simulink model "sdofDAEll_with_memory"  (R2023a)
settings: Solver=ode4  StartTime=0.0  StopTime=tmax  FixedStep=dt  RelTol=1e-3
InitFcn:
  | script_llm
values from neighbouring files (symbols this model uses):
  A1 = [O,I;-M1\K1,-M1\C1]    [script_llm.m]
  A2 = [O,I;-M2\K2,-M2\C2]    [script_llm.m]
  B1 = [0;0;M1\[0;1]]    [script_llm.m]
  B1b = -1    [script_llm.m]
  B2 = [0;0;M2\[0;1]]    [script_llm.m]
  B2b = -1    [script_llm.m]
  G1 = [0,0,0,1]    [script_llm.m]
  G1b = -1    [script_llm.m]
  G2 = [0,0,0,1]    [script_llm.m]
  G2b = -1    [script_llm.m]
  H1 = [0;0;0;1]    [script_llm.m]
  H2 = [0;0;0;0]    [script_llm.m]
settings Model: Creator=au621298  LastModifiedBy=Administrator

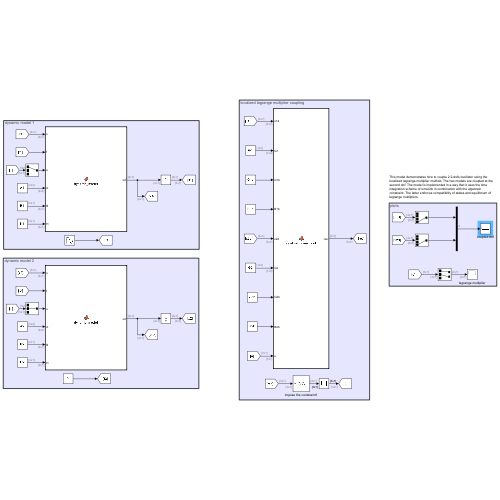
[thumbnail: Simulink's stored preview of the top-level diagram]
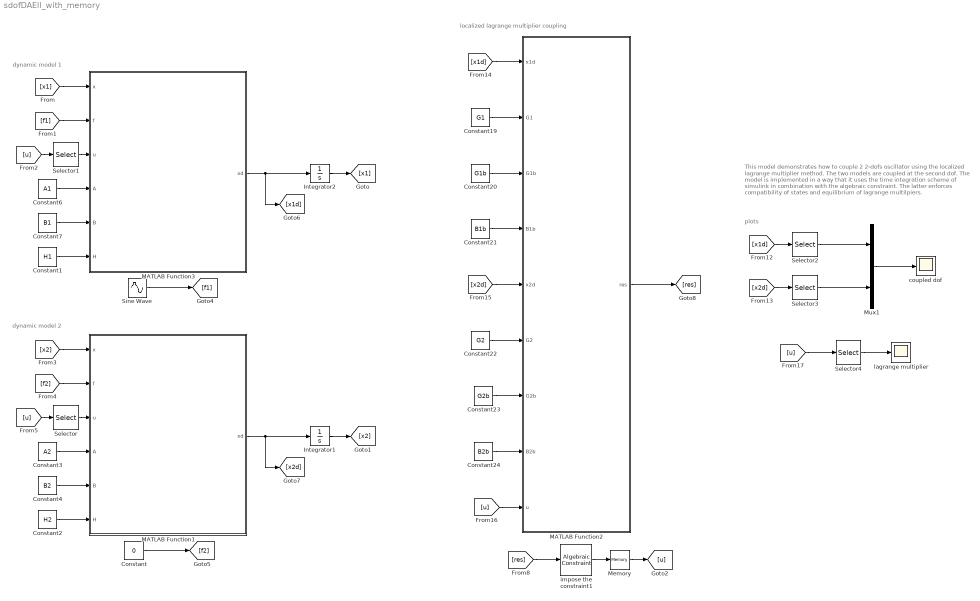
== system sdofDAEll_with_memory ==
  note: This model demonstrates how to couple 2 2-dofs oscillator using the localized lagrange multiplier method. The two models are coupled at the second dof. The model is implemented in a way that it uses the time integration scheme of simulink in combination with the algebraic constraint. The latter enforces compatibility of states and equilibrium of lagrange multilpiers.
  note: plots
  note: localized lagrange multiplier coupling
  note: dynamic model 2
  note: dynamic model 1
  Constant : Constant  Value=0
  Constant1 : Constant  Value=H1  VectorParams1D=off
  Constant19 : Constant  Value=G1  VectorParams1D=off
  Constant2 : Constant  Value=H2  VectorParams1D=off
  Constant20 : Constant  Value=G1b  VectorParams1D=off
  Constant21 : Constant  Value=B1b  VectorParams1D=off
  Constant22 : Constant  Value=G2  VectorParams1D=off
  Constant23 : Constant  Value=G2b  VectorParams1D=off
  Constant24 : Constant  Value=B2b  VectorParams1D=off
  Constant3 : Constant  Value=A2  VectorParams1D=off
  Constant4 : Constant  Value=B2  VectorParams1D=off
  Constant6 : Constant  Value=A1  VectorParams1D=off
  Constant7 : Constant  Value=B1  VectorParams1D=off
  Integrator1 : Integrator  InitialCondition=zeros(4,1)
  Integrator2 : Integrator  InitialCondition=zeros(4,1)
  MATLAB Function1 : MATLAB Function  TreatAsAtomicUnit=on
  MATLAB Function2 : MATLAB Function  TreatAsAtomicUnit=on
  MATLAB Function3 : MATLAB Function  TreatAsAtomicUnit=on
  Memory : Memory  InitialCondition=zeros(3,1)
  Mux1 : Mux  Inputs=2
  Selector : Selector  InputPortWidth=3  IndexOptions=Index vector (dialog)  Indices=2  OutputSizes=1
  Selector1 : Selector  InputPortWidth=3  IndexOptions=Index vector (dialog)  Indices=1  OutputSizes=1
  Selector2 : Selector  InputPortWidth=4  IndexOptions=Index vector (dialog)  Indices=4  OutputSizes=1
  Selector3 : Selector  InputPortWidth=4  IndexOptions=Index vector (dialog)  Indices=4  OutputSizes=1
  Selector4 : Selector  InputPortWidth=3  IndexOptions=Index vector (dialog)  Indices=[1,2]  OutputSizes=1
  Sine Wave : Sin  Amplitude=2  SampleTime=0
  coupled dof : Scope
  impose the constraint1 : AlgebraicConstraint
  lagrange multiplier : Scope
  wires:
  Constant6/1 -> MATLAB Function3/4(A)
  Constant7/1 -> MATLAB Function3/5(B)
  Mux1/1 -> coupled dof/1
  MATLAB Function3/1(xd) -> [x1d], Integrator2/1
  Selector2/1 -> Mux1/1
  Selector3/1 -> Mux1/2
  Constant1/1 -> MATLAB Function3/6(H)
  Integrator2/1 -> [x1]
  [x1] -> MATLAB Function3/1(x)
  [f1] -> MATLAB Function3/2(f)
  Constant2/1 -> MATLAB Function1/6(H)
  Constant4/1 -> MATLAB Function1/5(B)
  MATLAB Function1/1(xd) -> [x2d], Integrator1/1
  Constant3/1 -> MATLAB Function1/4(A)
  [x2] -> MATLAB Function1/1(x)
  [f2] -> MATLAB Function1/2(f)
  Integrator1/1 -> [x2]
  [u] -> Selector/1
  Selector/1 -> MATLAB Function1/3(u)
  Selector1/1 -> MATLAB Function3/3(u)
  [u] -> Selector1/1
  impose the constraint1/1 -> Memory/1
  [res] -> impose the constraint1/1
  Sine Wave/1 -> [f1]
  Constant/1 -> [f2]
  [x1d] -> Selector2/1
  [x2d] -> Selector3/1
  [x2d] -> MATLAB Function2/5(x2d)
  [x1d] -> MATLAB Function2/1(x1d)
  Constant19/1 -> MATLAB Function2/2(G1)
  Constant20/1 -> MATLAB Function2/3(G1b)
  Constant21/1 -> MATLAB Function2/4(B1b)
  Constant22/1 -> MATLAB Function2/6(G2)
  Constant23/1 -> MATLAB Function2/7(G2b)
  Constant24/1 -> MATLAB Function2/8(B2b)
  [u] -> MATLAB Function2/9(u)
  MATLAB Function2/1(res) -> [res]
  [u] -> Selector4/1
  Selector4/1 -> lagrange multiplier/1
  Memory/1 -> [u]

== matlab function sdofDAEll_with_memory/MATLAB Function1 ==
  data: x input; f input; u input; xd output; A input; B input; H input
function xd = dynamic_model(x,f,u,A,B,H)

% A1 = state transition matrix
% B = collocation matrix lagrange multipliers
% H = collocation matrix applied load
% x = state vector
% xd = state rate vector

xd = A*x + B*u + H*f;

end

== matlab function sdofDAEll_with_memory/MATLAB Function2 ==
  data: x1d input; G1 input; G1b input; B1b input; x2d input; res output; G2 input; G2b input; B2b input; u input
function res = algebraic_constraint(x1d,G1,G1b,B1b,x2d,G2,G2b,B2b,u)

u1 = u(1) ; % lagrange multiplier on model 1
u2 = u(2) ; % lagrange multiplier on model 2
xgd = u(3) ; % generalized interface dof

% res = [G1 * x1d + G1b * xgd ; % compatibility equation for model 1
%        G2 * x2d + G2b * xgd ; % compatibility equation for model 2
%        B1b*u1 + B2b*u2] ; % equilibrium of lagrange multipliers

res = [B1b*u1 + B2b*u2 ; % equilibrium of lagrange multipliers
       G1 * x1d + G1b * xgd ; % compatibility equation for model 1
       G2 * x2d + G2b * xgd] ; % compatibility equation for model 2
       

end

== matlab function sdofDAEll_with_memory/MATLAB Function3 ==
  data: x input; f input; u input; xd output; A input; B input; H input
function xd = dynamic_model(x,f,u,A,B,H)

% A1 = state transition matrix
% B = collocation matrix lagrange multipliers
% H = collocation matrix applied load
% x = state vector
% xd = state rate vector

xd = A*x + B*u + H*f;

end
